simulink model "W03_H_antiwindup"  (R2024b)
settings: Solver=ode4  StartTime=0  StopTime=aw_T  FixedStep=h  RelTol=1e-3
StopFcn:
  | W03_aw_plot;
undefined symbols (not defined in the file or in its folder): aw_Kb, aw_Ki, aw_Kp, aw_r1, aw_r2, aw_t1, aw_t2, aw_umax, aw_umin
libraries: slpidlib x3
settings Model: Creator=admin  LastModifiedBy=admin
settings DataIOCC: ReturnWorkspaceOutputs=off

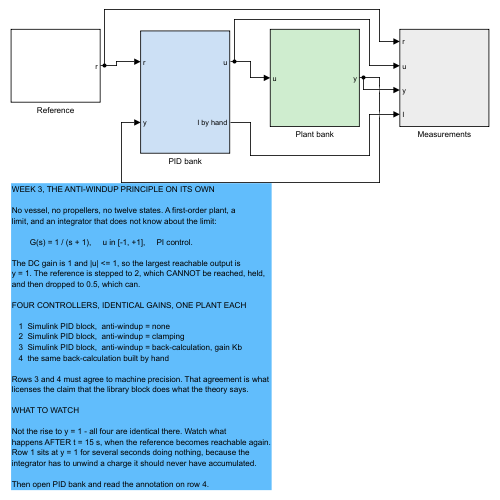
[thumbnail: Simulink's stored preview of the top-level diagram]
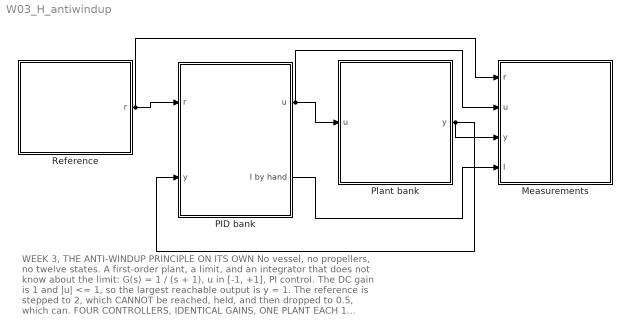
== system W03_H_antiwindup ==
  note: WEEK 3, THE ANTI-WINDUP PRINCIPLE ON ITS OWN
      |
      | No vessel, no propellers, no twelve states. A first-order plant, a
      | limit, and an integrator that does not know about the limit:
      |
      |         G(s) = 1 / (s + 1),     u in [-1, +1],     PI control.
      |
      | The DC gain is 1 and |u| <= 1, so the largest reachable output is
      | y = 1. The reference is stepped to 2, which CANNOT be reached, held,
      | and then dropped to 0.5, which can.
      |
      | FOUR CONTROLLERS, IDENTICAL GAINS, ONE PLANT EACH
      |
      |    1  Simulink PID block,  anti-windup = none
      |    2  Simulink PID block,  anti-windup = clamping
      |    3  Simulink PID block,  anti-windup = back-calculation, gain Kb
      |    4  the same back-calculation built by hand
      |
      | Rows 3 and 4 must agree to machine precision. That agreement is what
      | licenses the claim that the library block does what the theory says.
      |
      | WHAT TO WATCH
      |
      | Not the rise to y = 1 - all four are identical there. Watch what
      | happens AFTER t = 15 s, when the reference becomes reachable again.
      | Row 1 sits at y = 1 for several seconds doing nothing, because the
      | integrator has to unwind a charge it should never have accumulated.
      |
      | Then open PID bank and read the annotation on row 4.
  Measurements : Subsystem
  PID bank : Subsystem
  Plant bank : Subsystem
  Reference : Subsystem
  wires:
  Reference/1(r) -> PID bank/1(r), Measurements/1(r)
  Plant bank/1(y) -> PID bank/2(y), Measurements/3(y)
  PID bank/1(u) -> Plant bank/1(u), Measurements/2(u)
  PID bank/2(I by hand) -> Measurements/4(I)

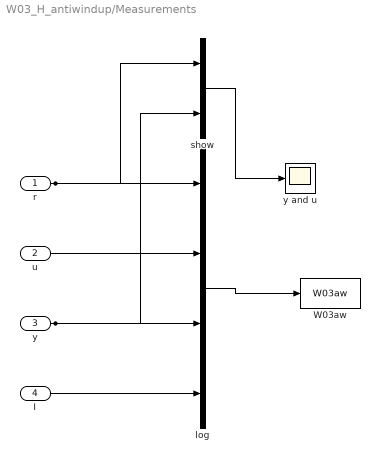
== system W03_H_antiwindup/Measurements ==
  r : Inport
  u : Inport  Port=2
  y : Inport  Port=3
  I : Inport  Port=4
  W03aw : ToWorkspace  VariableName=W03aw  SaveFormat=Structure With Time  SampleTime=-1
  log : Mux
  show : Mux  Inputs=2
  y and u : Scope
  wires:
  r/1 -> log/1, show/1
  u/1 -> log/2
  y/1 -> log/3, show/2
  I/1 -> log/4
  log/1 -> W03aw/1
  show/1 -> y and u/1

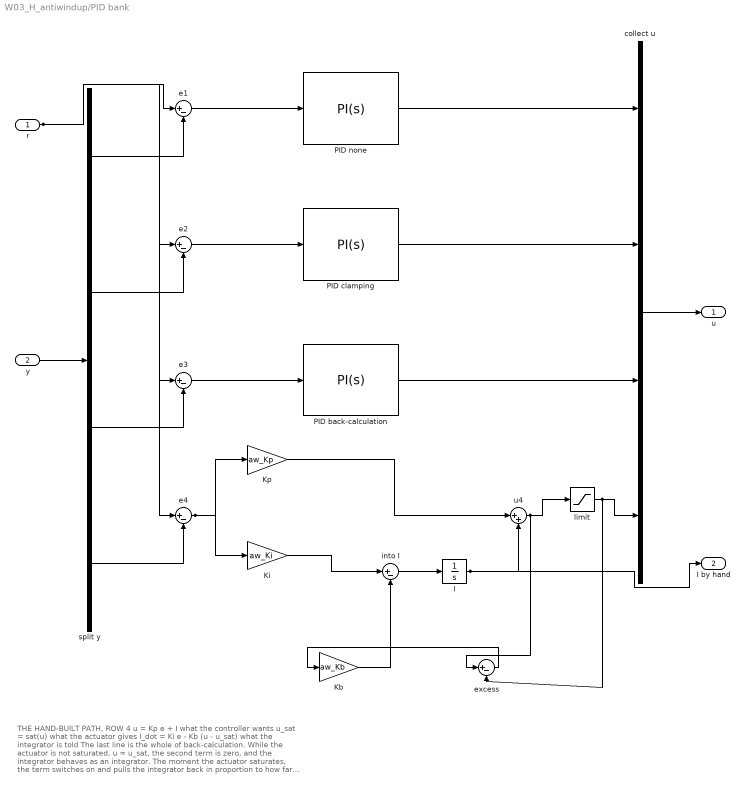
== system W03_H_antiwindup/PID bank ==
  note: THE HAND-BUILT PATH, ROW 4
      |
      |     u     = Kp e + I                 what the controller wants
      |     u_sat = sat(u)                   what the actuator gives
      |     I_dot = Ki e - Kb (u - u_sat)    what the integrator is told
      |
      | The last line is the whole of back-calculation. While the actuator is
      | not saturated, u = u_sat, the second term is zero, and the integrator
      | behaves as an integrator. The moment the actuator saturates, the term
      | switches on and pulls the integrator back in proportion to how far
      | outside the limit the demand has gone.
      |
      | Rows 3 and 4 must agree. If they do not, one of them is wrong.
  r : Inport
  y : Inport  Port=2
  I : Integrator
  Kb : Gain  Gain=aw_Kb
  Ki : Gain  Gain=aw_Ki
  Kp : Gain  Gain=aw_Kp
  PID back-calculation : slpidlib/PID Controller  Controller=PI  Form=Parallel  TimeDomain=Continuous-time  UseExternalTs=off  SampleTime=-1  IntegratorMethod=Forward Euler  FilterMethod=Forward Euler  ControllerParametersSource=internal  P=aw_Kp  I=aw_Ki  UseKiTs=off  D=0  UseExternalDerivativeSource=off  N=100  UseFilter=on  TunerSelectOption=Transfer Function Based (PID Tuner App)  InitialConditionSource=internal  InitialConditionForIntegrator=0  InitialConditionForFilter=0  DifferentiatorICPrevScaledInput=0  ExternalReset=none  TrackingMode=off  Kt=1  LimitOutput=on  SatLimitsSource=internal  UpperSaturationLimit=aw_umax  LowerSaturationLimit=aw_umin  LinearizeAsGain=on  AntiWindupMode=back-calculation  Kb=aw_Kb  LimitIntegrator=off  UpperIntegratorSaturationLimit=inf  LowerIntegratorSaturationLimit=-inf  POutMin=[]  POutMax=[]  IOutMin=[]  IOutMax=[]  DOutMin=[]  DOutMax=[]  NOutMin=[]  NOutMax=[]  SumOutMin=[]  SumOutMax=[]  SaturationOutMin=[]  SaturationOutMax=[]  PParamMin=[]  PParamMax=[]  IParamMin=[]  IParamMax=[]  DParamMin=[]  DParamMax=[]  NParamMin=[]  NParamMax=[]  KbParamMin=[]  KbParamMax=[]  KtParamMin=[]  KtParamMax=[]  KbOutMin=[]  KbOutMax=[]  KtOutMin=[]  KtOutMax=[]  IntegratorOutMin=[]  IntegratorOutMax=[]  FilterOutMin=[]  FilterOutMax=[]  SumI1OutMin=[]  SumI1OutMax=[]  SumI2OutMin=[]  SumI2OutMax=[]  SumI3OutMin=[]  SumI3OutMax=[]  SumI4OutMin=[]  SumI4OutMax=[]  SumDOutMin=[]  SumDOutMax=[]  DifferentiatorOutMin=[]  DifferentiatorOutMax=[]  FilterDiffOutCoefMin=[]  FilterDiffOutCoefMax=[]  ReciprocalOutMin=[]  ReciprocalOutMax=[]  SumDenOutMin=[]  SumDenOutMax=[]  SumNumOutMin=[]  SumNumOutMax=[]  DivideOutMin=[]  DivideOutMax=[]  UdiffTsProdOutMin=[]  UdiffTsProdOutMax=[]  NTsProdOutMin=[]  NTsProdOutMax=[]  UintegralTsProdOutMin=[]  UintegralTsProdOutMax=[]  UngainTsProdOutMin=[]  UngainTsProdOutMax=[]  ClampingZeroOutDataTypeStr=Inherit: Inherit via back propagation  ClampingZeroOutMin=[]  ClampingZeroOutMax=[]  FilterDenConstantOutDataTypeStr=Inherit: Inherit via back propagation  FilterDenConstantOutMin=[]  FilterDenConstantOutMax=[]  PCopyOutDataTypeStr=Inherit: Inherit via back propagation  PCopyOutMin=[]  PCopyOutMax=[]  NCopyOutDataTypeStr=Inherit: Inherit via back propagation  NCopyOutMin=[]  NCopyOutMax=[]  IntegratorContinuousStateAttributes=''  IntegratorStateMustResolveToSignalObject=off  IntegratorRTWStateStorageClass=Auto  FilterContinuousStateAttributes=''  FilterStateMustResolveToSignalObject=off  FilterRTWStateStorageClass=Auto  ParallelPVariant=InternalParameters  IdealPVariant=Disabled  IVariant=InternalParameters  DVariant=Disabled  IntegratorVariant=Continuous  SatVariant=Enabled  AWVariant=BackCalculation  PCopyVariant=Disabled  TRVariant=Disabled  FdbkBlocksVariant=Forward  IdealPFdbkVariant=Disabled  SatFdbkVariant=Disabled  DerivativeFilterVariant=Disabled  NVariant=Disabled  NCopyVariant=Disabled_SignalSpec  FilterICVariant=Disabled  IntegratorICVariant=InternalICs  ExternalResetVariant=Disabled  TRSumVariant=Passthrough  SumFdbkVariant=Disabled  SumVariant=Sum_PI  TsampFilterVariant=InternalTs  TsampNgainVariant=Passthrough  TsampIntegralVariant=Disabled_SignalSpec  ExternalSaturationOutDataTypeStr=Inherit: Same as second input  DerivativeSourceVariant=Disabled  PreIntVariant=InternalPreInt
  PID clamping : slpidlib/PID Controller  Controller=PI  Form=Parallel  TimeDomain=Continuous-time  UseExternalTs=off  SampleTime=-1  IntegratorMethod=Forward Euler  FilterMethod=Forward Euler  ControllerParametersSource=internal  P=aw_Kp  I=aw_Ki  UseKiTs=off  D=0  UseExternalDerivativeSource=off  N=100  UseFilter=on  TunerSelectOption=Transfer Function Based (PID Tuner App)  InitialConditionSource=internal  InitialConditionForIntegrator=0  InitialConditionForFilter=0  DifferentiatorICPrevScaledInput=0  ExternalReset=none  TrackingMode=off  Kt=1  LimitOutput=on  SatLimitsSource=internal  UpperSaturationLimit=aw_umax  LowerSaturationLimit=aw_umin  LinearizeAsGain=on  AntiWindupMode=clamping  Kb=aw_Kb  LimitIntegrator=off  UpperIntegratorSaturationLimit=inf  LowerIntegratorSaturationLimit=-inf  POutMin=[]  POutMax=[]  IOutMin=[]  IOutMax=[]  DOutMin=[]  DOutMax=[]  NOutMin=[]  NOutMax=[]  SumOutMin=[]  SumOutMax=[]  SaturationOutMin=[]  SaturationOutMax=[]  PParamMin=[]  PParamMax=[]  IParamMin=[]  IParamMax=[]  DParamMin=[]  DParamMax=[]  NParamMin=[]  NParamMax=[]  KbParamMin=[]  KbParamMax=[]  KtParamMin=[]  KtParamMax=[]  KbOutMin=[]  KbOutMax=[]  KtOutMin=[]  KtOutMax=[]  IntegratorOutMin=[]  IntegratorOutMax=[]  FilterOutMin=[]  FilterOutMax=[]  SumI1OutMin=[]  SumI1OutMax=[]  SumI2OutMin=[]  SumI2OutMax=[]  SumI3OutMin=[]  SumI3OutMax=[]  SumI4OutMin=[]  SumI4OutMax=[]  SumDOutMin=[]  SumDOutMax=[]  DifferentiatorOutMin=[]  DifferentiatorOutMax=[]  FilterDiffOutCoefMin=[]  FilterDiffOutCoefMax=[]  ReciprocalOutMin=[]  ReciprocalOutMax=[]  SumDenOutMin=[]  SumDenOutMax=[]  SumNumOutMin=[]  SumNumOutMax=[]  DivideOutMin=[]  DivideOutMax=[]  UdiffTsProdOutMin=[]  UdiffTsProdOutMax=[]  NTsProdOutMin=[]  NTsProdOutMax=[]  UintegralTsProdOutMin=[]  UintegralTsProdOutMax=[]  UngainTsProdOutMin=[]  UngainTsProdOutMax=[]  ClampingZeroOutDataTypeStr=Inherit: Inherit via back propagation  ClampingZeroOutMin=[]  ClampingZeroOutMax=[]  FilterDenConstantOutDataTypeStr=Inherit: Inherit via back propagation  FilterDenConstantOutMin=[]  FilterDenConstantOutMax=[]  PCopyOutDataTypeStr=Inherit: Inherit via back propagation  PCopyOutMin=[]  PCopyOutMax=[]  NCopyOutDataTypeStr=Inherit: Inherit via back propagation  NCopyOutMin=[]  NCopyOutMax=[]  IntegratorContinuousStateAttributes=''  IntegratorStateMustResolveToSignalObject=off  IntegratorRTWStateStorageClass=Auto  FilterContinuousStateAttributes=''  FilterStateMustResolveToSignalObject=off  FilterRTWStateStorageClass=Auto  ParallelPVariant=InternalParameters  IdealPVariant=Disabled  IVariant=InternalParameters  DVariant=Disabled  IntegratorVariant=Continuous  SatVariant=Enabled  AWVariant=ContClampingParallel  PCopyVariant=Disabled  TRVariant=Disabled  FdbkBlocksVariant=Forward  IdealPFdbkVariant=Disabled  SatFdbkVariant=Disabled  DerivativeFilterVariant=Disabled  NVariant=Disabled  NCopyVariant=Disabled_SignalSpec  FilterICVariant=Disabled  IntegratorICVariant=InternalICs  ExternalResetVariant=Disabled  TRSumVariant=Passthrough  SumFdbkVariant=Disabled  SumVariant=Sum_PI  TsampFilterVariant=InternalTs  TsampNgainVariant=Passthrough  TsampIntegralVariant=Disabled_SignalSpec  ExternalSaturationOutDataTypeStr=Inherit: Same as second input  DerivativeSourceVariant=Disabled  PreIntVariant=InternalPreInt
  PID none : slpidlib/PID Controller  Controller=PI  Form=Parallel  TimeDomain=Continuous-time  UseExternalTs=off  SampleTime=-1  IntegratorMethod=Forward Euler  FilterMethod=Forward Euler  ControllerParametersSource=internal  P=aw_Kp  I=aw_Ki  UseKiTs=off  D=0  UseExternalDerivativeSource=off  N=100  UseFilter=on  TunerSelectOption=Transfer Function Based (PID Tuner App)  InitialConditionSource=internal  InitialConditionForIntegrator=0  InitialConditionForFilter=0  DifferentiatorICPrevScaledInput=0  ExternalReset=none  TrackingMode=off  Kt=1  LimitOutput=on  SatLimitsSource=internal  UpperSaturationLimit=aw_umax  LowerSaturationLimit=aw_umin  LinearizeAsGain=on  AntiWindupMode=none  Kb=aw_Kb  LimitIntegrator=off  UpperIntegratorSaturationLimit=inf  LowerIntegratorSaturationLimit=-inf  POutMin=[]  POutMax=[]  IOutMin=[]  IOutMax=[]  DOutMin=[]  DOutMax=[]  NOutMin=[]  NOutMax=[]  SumOutMin=[]  SumOutMax=[]  SaturationOutMin=[]  SaturationOutMax=[]  PParamMin=[]  PParamMax=[]  IParamMin=[]  IParamMax=[]  DParamMin=[]  DParamMax=[]  NParamMin=[]  NParamMax=[]  KbParamMin=[]  KbParamMax=[]  KtParamMin=[]  KtParamMax=[]  KbOutMin=[]  KbOutMax=[]  KtOutMin=[]  KtOutMax=[]  IntegratorOutMin=[]  IntegratorOutMax=[]  FilterOutMin=[]  FilterOutMax=[]  SumI1OutMin=[]  SumI1OutMax=[]  SumI2OutMin=[]  SumI2OutMax=[]  SumI3OutMin=[]  SumI3OutMax=[]  SumI4OutMin=[]  SumI4OutMax=[]  SumDOutMin=[]  SumDOutMax=[]  DifferentiatorOutMin=[]  DifferentiatorOutMax=[]  FilterDiffOutCoefMin=[]  FilterDiffOutCoefMax=[]  ReciprocalOutMin=[]  ReciprocalOutMax=[]  SumDenOutMin=[]  SumDenOutMax=[]  SumNumOutMin=[]  SumNumOutMax=[]  DivideOutMin=[]  DivideOutMax=[]  UdiffTsProdOutMin=[]  UdiffTsProdOutMax=[]  NTsProdOutMin=[]  NTsProdOutMax=[]  UintegralTsProdOutMin=[]  UintegralTsProdOutMax=[]  UngainTsProdOutMin=[]  UngainTsProdOutMax=[]  ClampingZeroOutDataTypeStr=Inherit: Inherit via back propagation  ClampingZeroOutMin=[]  ClampingZeroOutMax=[]  FilterDenConstantOutDataTypeStr=Inherit: Inherit via back propagation  FilterDenConstantOutMin=[]  FilterDenConstantOutMax=[]  PCopyOutDataTypeStr=Inherit: Inherit via back propagation  PCopyOutMin=[]  PCopyOutMax=[]  NCopyOutDataTypeStr=Inherit: Inherit via back propagation  NCopyOutMin=[]  NCopyOutMax=[]  IntegratorContinuousStateAttributes=''  IntegratorStateMustResolveToSignalObject=off  IntegratorRTWStateStorageClass=Auto  FilterContinuousStateAttributes=''  FilterStateMustResolveToSignalObject=off  FilterRTWStateStorageClass=Auto  ParallelPVariant=InternalParameters  IdealPVariant=Disabled  IVariant=InternalParameters  DVariant=Disabled  IntegratorVariant=Continuous  SatVariant=Enabled  AWVariant=Passthrough  PCopyVariant=Disabled  TRVariant=Disabled  FdbkBlocksVariant=Forward  IdealPFdbkVariant=Disabled  SatFdbkVariant=Disabled  DerivativeFilterVariant=Disabled  NVariant=Disabled  NCopyVariant=Disabled_SignalSpec  FilterICVariant=Disabled  IntegratorICVariant=InternalICs  ExternalResetVariant=Disabled  TRSumVariant=Passthrough  SumFdbkVariant=Disabled  SumVariant=Sum_PI  TsampFilterVariant=InternalTs  TsampNgainVariant=Passthrough  TsampIntegralVariant=Disabled_SignalSpec  ExternalSaturationOutDataTypeStr=Inherit: Same as second input  DerivativeSourceVariant=Disabled  PreIntVariant=InternalPreInt
  collect u : Mux
  e{1..4} (4 alike) : Sum  Inputs=|+-
  excess : Sum  Inputs=|+-
  into I : Sum  Inputs=|+-
  limit : Saturate  UpperLimit=aw_umax  LowerLimit=aw_umin
  split y : Demux
  u4 : Sum  Inputs=|++
  u : Outport
  I by hand : Outport  Port=2
  wires:
  y/1 -> split y/1
  collect u/1 -> u/1
  r/1 -> e1/1, e2/1, e3/1, e4/1
  split y/1 -> e1/2
  e1/1 -> PID none/1
  PID none/1 -> collect u/1
  split y/2 -> e2/2
  e2/1 -> PID clamping/1
  PID clamping/1 -> collect u/2
  split y/3 -> e3/2
  e3/1 -> PID back-calculation/1
  PID back-calculation/1 -> collect u/3
  split y/4 -> e4/2
  e4/1 -> Kp/1, Ki/1
  Ki/1 -> into I/1
  Kb/1 -> into I/2
  into I/1 -> I/1
  Kp/1 -> u4/1
  I/1 -> u4/2, I by hand/1
  u4/1 -> limit/1, excess/1
  limit/1 -> excess/2, collect u/4
  excess/1 -> Kb/1

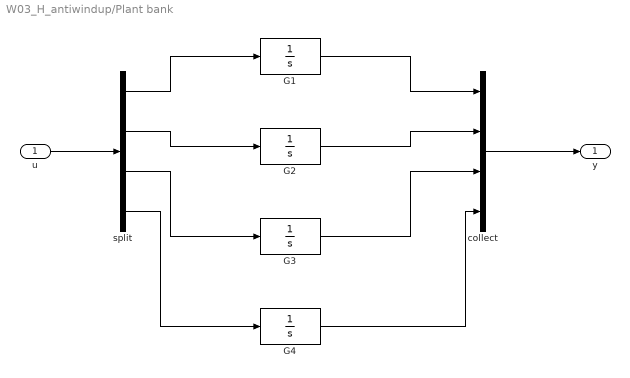
== system W03_H_antiwindup/Plant bank ==
  u : Inport
  G{1..4} (4 alike) : TransferFcn  Denominator=[1 0]
  collect : Mux
  split : Demux
  y : Outport
  wires:
  u/1 -> split/1
  collect/1 -> y/1
  split/1 -> G1/1
  G1/1 -> collect/1
  split/2 -> G2/1
  G2/1 -> collect/2
  split/3 -> G3/1
  G3/1 -> collect/3
  split/4 -> G4/1
  G4/1 -> collect/4

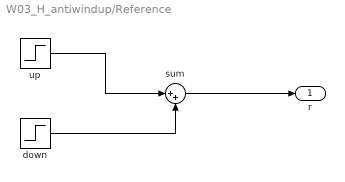
== system W03_H_antiwindup/Reference ==
  down : Step  Time=aw_t2  After=aw_r2 - aw_r1  SampleTime=0
  sum : Sum  Inputs=|++
  up : Step  Time=aw_t1  After=aw_r1  SampleTime=0
  r : Outport
  wires:
  up/1 -> sum/1
  down/1 -> sum/2
  sum/1 -> r/1
